simulink model "Final_Project"  (R2021a)
settings: Solver=VariableStepAuto  StartTime=0.0  StopTime=10.0  RelTol=1e-3
libraries: spsSeriesRLCBranchLib x3, spsCurrentMeasurementLib x2, dspstat3 x2, spsVoltageMeasurementLib x2, spsFirstOrderFilterLib x1, spsPermanentMagnetSynchronousMachineLib x1, simulink x1, spsThreePhaseVIMeasurementLib x1, spsUniversalBridgeLib x1, spsWindTurbineLib x1
settings Model: Creator=Sourav Das  LastModifiedBy=Sourav Das

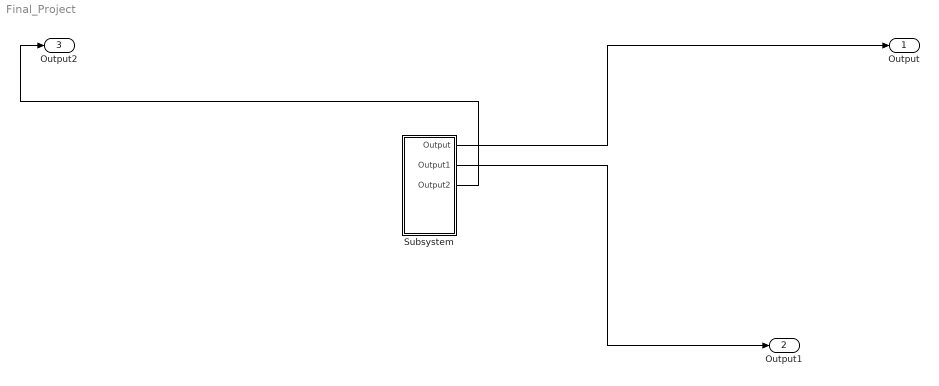
== system Final_Project ==
  Subsystem : Subsystem
  Output : Outport
  Output1 : Outport  Port=2
  Output2 : Outport  Port=3
  wires:
  Subsystem/1(Output) -> Output/1
  Subsystem/2(Output1) -> Output1/1
  Subsystem/3(Output2) -> Output2/1

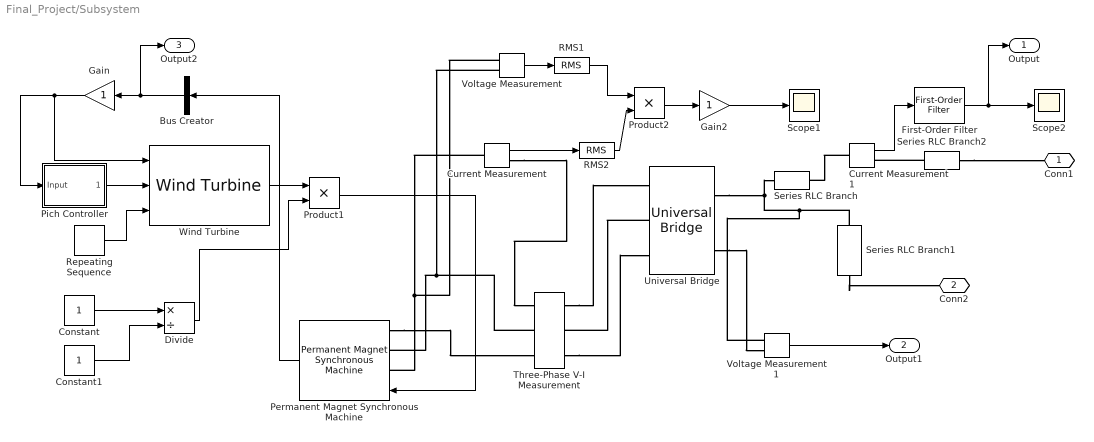
== system Final_Project/Subsystem ==
  Bus Creator : BusCreator  Inputs=1
  Constant : Constant
  Constant1 : Constant
  Current Measurement : spsCurrentMeasurementLib/Current Measurement  PhasorSimulation=off  OutputType=Complex  PSBequivalent=0
  Current Measurement1 : spsCurrentMeasurementLib/Current Measurement  PhasorSimulation=off  OutputType=Complex  PSBequivalent=0
  Divide : Product  Inputs=*/
  First-Order Filter : spsFirstOrderFilterLib/First-Order Filter  FilterType=Lowpass  Tc=10e-3  Ts=0  Initialize=on  Vac_Init=[0, 0, 60]  Vdc_Init=0  PlotResponse=off  FreqRange="[0,  200,  1]"
  Gain : Gain
  Gain2 : Gain
  Permanent Magnet Synchronous Machine : spsPermanentMagnetSynchronousMachineLib/Permanent Magnet Synchronous Machine  NbPhases=3  FluxDistribution=Sinusoidal  RotorType=Round  MechanicalLoad=Torque Tm  PresetModel=No  ShowDetailedParameters=on  MeasurementBus=off  Resistance=0.0485  Inductance=8.5e-3  dqInductances=[8.5e-3,8.5e-3]  La=0.000395  MachineConstant=Flux linkage established by magnets (V.s)  Flux=0.1194  VoltageCst=86.6271  TorqueCst=0.7164  Flat=120  Mechanical=[0.0027 0.0004924 4 0]  PolePairs=4  InitialConditions=[0,0, 0,0]  InitialConditions5ph=[0 0 0 0 0 0]  RefAngle=90 degrees behind phase A axis (modified Park)  IterativeDiscreteModel=Trapezoidal non iterative  TsBlock=-1  TsPowergui=0
  Pich Controller : Subsystem
  Product1 : Product
  Product2 : Product
  RMS1 : dspstat3/RMS  run=off  directionMode=Each column  dimension=1  InputProcessing=Columns as channels (frame based)  reset_popup=None
  RMS2 : dspstat3/RMS  run=off  directionMode=Each column  dimension=1  InputProcessing=Columns as channels (frame based)  reset_popup=None
  Repeating Sequence : simulink/Sources/Repeating Sequence  rep_seq_t=[0 2]  rep_seq_y=[0 2]
  Scope1 : Scope
  Scope2 : Scope
  Series RLC Branch : spsSeriesRLCBranchLib/Series RLC Branch  LConnTagsString=__new0  RConnTagsString=__new0  BranchType=L  Resistance=1  Inductance=1e-3  SetiL0=off  InitialCurrent=0  Capacitance=1e-6  Setx0=off  InitialVoltage=0  Measurements=None
  Series RLC Branch1 : spsSeriesRLCBranchLib/Series RLC Branch  LConnTagsString=__new0  RConnTagsString=__new0  BranchType=C  Resistance=1  Inductance=1e-3  SetiL0=off  InitialCurrent=0  Capacitance=1e-6  Setx0=off  InitialVoltage=0  Measurements=None
  Series RLC Branch2 : spsSeriesRLCBranchLib/Series RLC Branch  LConnTagsString=__new0  RConnTagsString=__new0  BranchType=L  Resistance=1  Inductance=1e-3  SetiL0=off  InitialCurrent=0  Capacitance=1e-6  Setx0=off  InitialVoltage=0  Measurements=None
  Three-Phase V-I Measurement : spsThreePhaseVIMeasurementLib/Three-Phase V-I Measurement  VoltageMeasurement=no  SetLabelV=off  LabelV=Vabc  Vpu=off  VpuLL=off  CurrentMeasurement=no  SetLabelI=off  LabelI=Iabc  Ipu=off  Pbase=100e6  Vbase=500e3  OutputType=Complex  PhasorSimulation=off  PSBequivalent=0
  Universal Bridge : spsUniversalBridgeLib/Universal Bridge  Arms=3  SnubberResistance=1e5  SnubberCapacitance=inf  Device=Diodes  Ron=1e-3  Lon=0  ForwardVoltages="[  0  0  ]"  ForwardVoltage=0  GTOparameters=[ 10e-6 , 20e-6 ]  IGBTparameters=[ 1e-6 , 2e-6 ]  Measurements=None  Measurements_2=None  converterType=Rectifier
  Voltage Measurement : spsVoltageMeasurementLib/Voltage Measurement  PhasorSimulation=off  OutputType=Complex  PSBequivalent=0
  Voltage Measurement1 : spsVoltageMeasurementLib/Voltage Measurement  PhasorSimulation=off  OutputType=Complex  PSBequivalent=0
  Wind Turbine : spsWindTurbineLib/Wind Turbine  Pnom=1.5e6  Pelec_base=1.5e6/0.9  wind_base=12  P_wind_base=0.73  speed_nom=1.2  pitch_angle=0  c1_c6="[0.51763          116          0.4            5           21     0.006795]"  cp_nom=0.48  lambda_nom=8.1
      settings: SourceProductBaseCode=PS
  Conn1 : PMIOPort  Side=Right
  Conn2 : PMIOPort  Port=2  Side=Right
  Output : Outport
  Output1 : Outport  Port=2
  Output2 : Outport  Port=3
  wires:
  First-Order Filter/1 -> Output/1, Scope2/1
  Gain/1 -> Wind Turbine/1, Pich Controller/1(Input)
  Current Measurement/1 -> RMS2/1
  Product1/1 -> Permanent Magnet Synchronous Machine/1
  Current Measurement1/1 -> First-Order Filter/1
  Repeating Sequence/1 -> Wind Turbine/3
  Voltage Measurement/1 -> RMS1/1
  Pich Controller/1(Output) -> Wind Turbine/2
  Voltage Measurement1/1 -> Output1/1
  Bus Creator/1 -> Output2/1, Gain/1
  Wind Turbine/1 -> Product1/1
  Product2/1 -> Gain2/1
  Constant1/1 -> Divide/2
  RMS2/1 -> Product2/2
  Permanent Magnet Synchronous Machine/1 -> Bus Creator/1
  Constant/1 -> Divide/1
  Divide/1 -> Product1/2
  RMS1/1 -> Product2/1
  Gain2/1 -> Scope1/1
  connections:
  Voltage Measurement/LConn2 -- Permanent Magnet Synchronous Machine/LConn2 -- Three-Phase V-I Measurement/LConn2
  Voltage Measurement/LConn1 -- Current Measurement/LConn1 -- Permanent Magnet Synchronous Machine/LConn1
  Current Measurement1/LConn1 -- Series RLC Branch/RConn1
  Universal Bridge/LConn2 -- Three-Phase V-I Measurement/RConn2
  Three-Phase V-I Measurement/RConn3 -- Universal Bridge/LConn3
  Three-Phase V-I Measurement/RConn1 -- Universal Bridge/LConn1
  Permanent Magnet Synchronous Machine/LConn3 -- Three-Phase V-I Measurement/LConn3
  Universal Bridge/RConn1 -- Series RLC Branch/LConn1 -- Voltage Measurement1/LConn1 -- Series RLC Branch1/LConn1
  Series RLC Branch2/RConn1 -- Conn1/RConn1
  Current Measurement/RConn1 -- Three-Phase V-I Measurement/LConn1
  Universal Bridge/RConn2 -- Voltage Measurement1/LConn2
  Series RLC Branch2/LConn1 -- Current Measurement1/RConn1
  Series RLC Branch1/RConn1 -- Conn2/RConn1

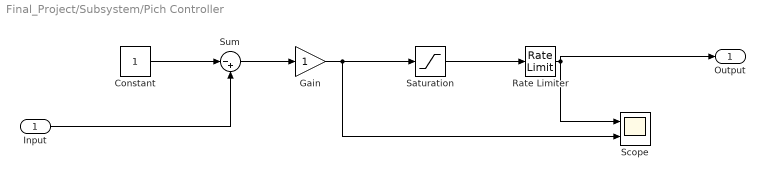
== system Final_Project/Subsystem/Pich Controller ==
  Input : Inport
  Constant : Constant
  Gain : Gain
  Rate Limiter : RateLimiter  SampleTimeMode=inherited
  Saturation : Saturate
  Scope : Scope  NumInputPorts=2
  Sum : Sum  Inputs=|-+
  Output : Outport
  wires:
  Saturation/1 -> Rate Limiter/1
  Rate Limiter/1 -> Output/1, Scope/1
  Constant/1 -> Sum/1
  Sum/1 -> Gain/1
  Gain/1 -> Scope/2, Saturation/1
  Input/1 -> Sum/2
